simulink library "sensor_processing_fsw_lib"  (R2016b)
settings: Solver=VariableStepAuto  StartTime=0.0  StopTime=10.0  RelTol=1e-3
libraries: sensor_processing_libs x2
settings Model: Creator=taylorreynolds  LastModifiedBy=taylorreynolds

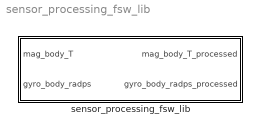
== system sensor_processing_fsw_lib ==
  sensor_processing_fsw_lib : Subsystem

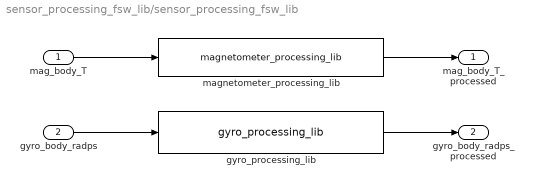
== system sensor_processing_fsw_lib/sensor_processing_fsw_lib ==
  mag_body_T : Inport
  gyro_body_radps : Inport  Port=2
  gyro_processing_lib : sensor_processing_libs/gyro_processing_lib
  magnetometer_processing_lib : sensor_processing_libs/magnetometer_processing_lib
  mag_body_T_processed : Outport
  gyro_body_radps_processed : Outport  Port=2
  wires:
  mag_body_T/1 -> magnetometer_processing_lib/1
  magnetometer_processing_lib/1 -> mag_body_T_processed/1
  gyro_body_radps/1 -> gyro_processing_lib/1
  gyro_processing_lib/1 -> gyro_body_radps_processed/1
